simulink model "SecondOrderUnderdampedSystem"  (R2023b)
settings: Solver=VariableStepAuto  StartTime=0.0  StopTime=20  RelTol=1e-3
values from neighbouring files (symbols this model uses):
  G_den = [A C E G I A]    [SecondOrderUnderdampedSystem_NonlinearSystemApproximation.m]    (also in SecondOrderUnderdampedSystem_NonlinearSystemApproximation_.m)
  G_num = [J H F D B]    [SecondOrderUnderdampedSystem_NonlinearSystemApproximation.m]    (also in SecondOrderUnderdampedSystem_NonlinearSystemApproximation_.m)
settings Model: Creator=gelibean  LastModifiedBy=gelibean

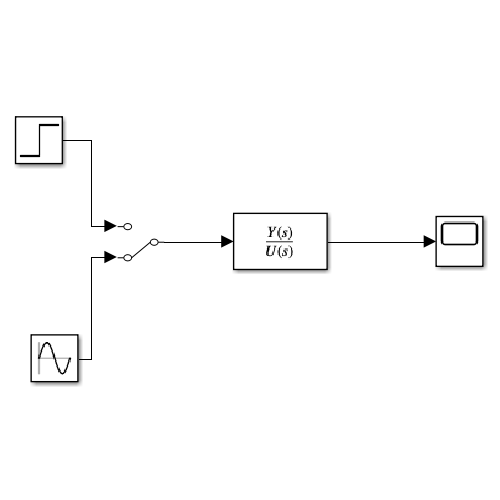
[thumbnail: Simulink's stored preview of the top-level diagram]
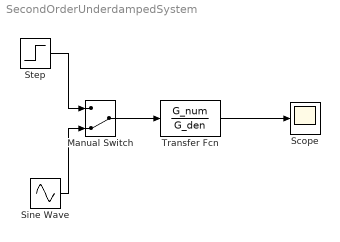
== system SecondOrderUnderdampedSystem ==
  Manual Switch : ManualSwitch  CurrentSetting=0
  Scope : Scope
  Sine Wave : Sin  SampleTime=0
  Step : Step  Time=0  SampleTime=0
  Transfer Fcn : TransferFcn  Numerator=G_num  Denominator=G_den
  wires:
  Transfer Fcn/1 -> Scope/1
  Manual Switch/1 -> Transfer Fcn/1
  Sine Wave/1 -> Manual Switch/2
  Step/1 -> Manual Switch/1
